simulink model "e_Ultrasonic"  (R2015a)
settings: Solver=ode45  StartTime=0.0  StopTime=10.0  RelTol=1e-3
settings Model: Creator=mattia  LastModifiedBy=pela

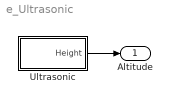
== system e_Ultrasonic ==
  Ultrasonic : Subsystem
  Altitude : Outport
  wires:
  Ultrasonic/1(Height) -> Altitude/1

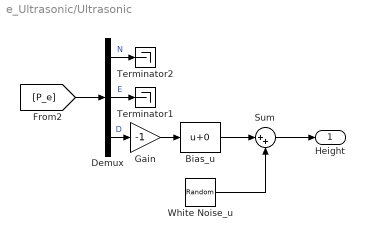
== system e_Ultrasonic/Ultrasonic ==
  Bias_u : Bias
  Demux : Demux  Outputs=3
  Gain : Gain  Gain=-1
  Sum : Sum  Inputs=|++
  Terminator1 : Terminator
  Terminator2 : Terminator
  White Noise_u : RandomNumber  DisableCoverage=on  Variance=0.00001  SampleTime=0.01
  Height : Outport
  wires:
  Sum/1 -> Height/1
  Demux/2 -> Terminator1/1  "E"
  [P_e] -> Demux/1
  Bias_u/1 -> Sum/1
  White Noise_u/1 -> Sum/2
  Demux/3 -> Gain/1  "D"
  Demux/1 -> Terminator2/1  "N"
  Gain/1 -> Bias_u/1
